simulink model "Exemplo2_Simulink"  (R2016a)
settings: Solver=VariableStepAuto  SolverMode=SingleTasking  StartTime=0.0  StopTime=10.0  RelTol=1e-3
values from neighbouring files (symbols this model uses):
  G1d = [1 1]    [Exemplo2.m]
  G1n = 1    [Exemplo2.m]
  G2d = [1 10 29]    [Exemplo2.m]
  G2n = 1    [Exemplo2.m]
  G3d = [1 0]    [Exemplo2.m]
  G3n = -5    [Exemplo2.m]
  G4d = 1    [Exemplo2.m]
  G4n = 10    [Exemplo2.m]
  G5d = 1    [Exemplo2.m]
  G5n = 25    [Exemplo2.m]
  G6d = [1 0]    [Exemplo2.m]
  G6n = -1    [Exemplo2.m]
  Gd = G.Denominator{1}    [Exemplo2.m]
  Gn = G.Numerator{1}    [Exemplo2.m]
settings Model: Creator=rafae  LastModifiedBy=rafae
settings DataIOCC: ReturnWorkspaceOutputs=on
settings DebuggingCC: SFUnexpectedBacktrackingDiag=error  SFNoUnconditionalDefaultTransitionDiag=error
settings SFSimCC: SimUseLocalCustomCode=on
settings RTWCC: RTWUseLocalCustomCode=on
settings GRTTargetCC: TargetLangStandard=C99 (ISO)
settings ConfigComp: CovMetricSettings=dwe  CovSaveCumulativeToWorkspaceVar=off  CovSaveSingleToWorkspaceVar=off  CovExternalEMLEnable=on

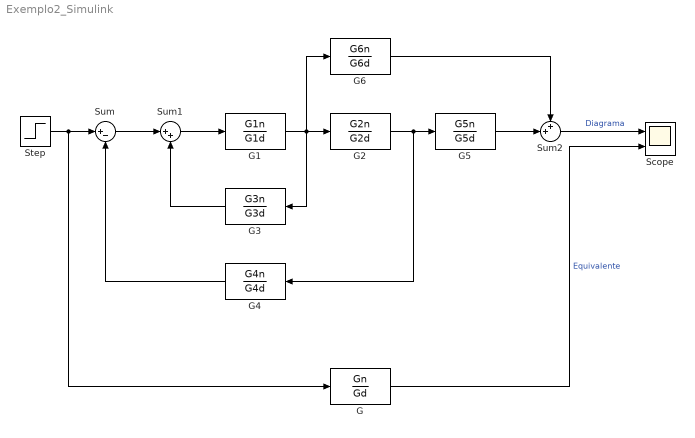
== system Exemplo2_Simulink ==
  G : TransferFcn  Numerator=Gn  Denominator=Gd
  G1 : TransferFcn  Numerator=G1n  Denominator=G1d
  G2 : TransferFcn  Numerator=G2n  Denominator=G2d
  G3 : TransferFcn  Numerator=G3n  Denominator=G3d
  G4 : TransferFcn  Numerator=G4n  Denominator=G4d
  G5 : TransferFcn  Numerator=G5n  Denominator=G5d
  G6 : TransferFcn  Numerator=G6n  Denominator=G6d
  Scope : Scope  NumInputPorts=2
  Step : Step  SampleTime=0
  Sum : Sum  Inputs=|+-
  Sum1 : Sum  Inputs=|++
  Sum2 : Sum  Inputs=++|
  wires:
  Sum/1 -> Sum1/1
  G2/1 -> G4/1, G5/1
  Sum1/1 -> G1/1
  G1/1 -> G6/1, G3/1, G2/1
  G6/1 -> Sum2/1
  G5/1 -> Sum2/2
  G3/1 -> Sum1/2
  Step/1 -> G/1, Sum/1
  G4/1 -> Sum/2
  Sum2/1 -> Scope/1  "Diagrama"
  G/1 -> Scope/2  "Equivalente"
